simulink model "model31"  (R2024a)
settings: Solver=VariableStepAuto  StartTime=0.0  StopTime=10.0  RelTol=1e-5
values from neighbouring files (symbols this model uses):
  k = kVal(i)    [script31.m]    (also in script32.m)
settings Model: Creator=eva  LastModifiedBy=eva

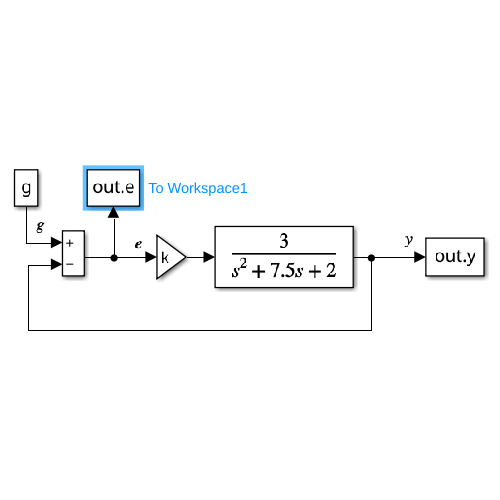
[thumbnail: Simulink's stored preview of the top-level diagram]
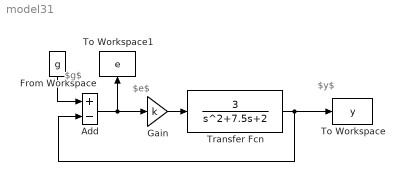
== system model31 ==
  note: $y$
  note: $g$
  note: $e$
  Add : Sum  Inputs=+-
  From Workspace : FromWorkspace  VariableName=g
  Gain : Gain  Gain=k
  To Workspace : ToWorkspace  VariableName=y  SaveFormat=Structure With Time  SampleTime=-1
  To Workspace1 : ToWorkspace  VariableName=e  SaveFormat=Structure With Time  SampleTime=-1
  Transfer Fcn : TransferFcn  Numerator=[3]  Denominator=[1 7.5 2]
  wires:
  Gain/1 -> Transfer Fcn/1
  Transfer Fcn/1 -> To Workspace/1, Add/2
  From Workspace/1 -> Add/1
  Add/1 -> To Workspace1/1, Gain/1
